simulink model "circuit5"  (Simulink 5.0)
settings: Solver=ode23tb  StartTime=0.0  StopTime=1  FixedStep=10e-6  RelTol=1e-4
undefined symbols (not defined in the file): A, powericon
libraries: powerlib2 x8, powerlib_extras x3, powerlib_models x1
settings Model: LastModifiedBy=Администратор

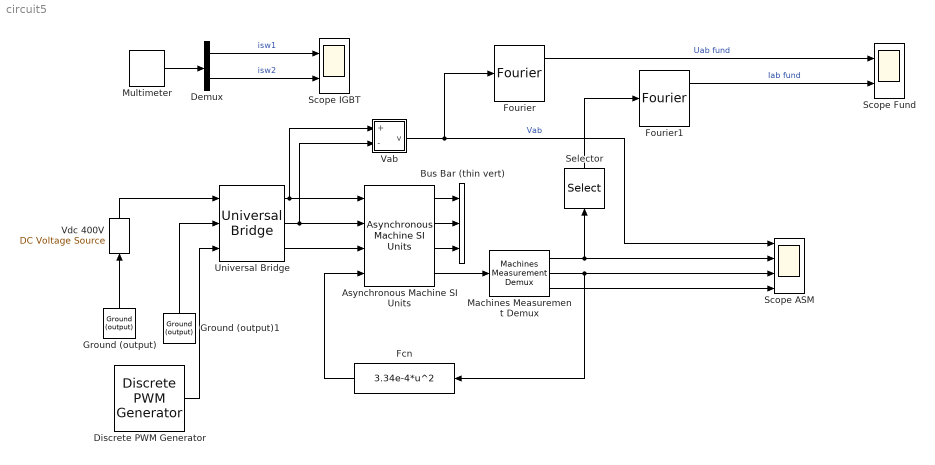
== system circuit5 ==
  Asynchronous Machine SI Units : powerlib2/Machines/Asynchronous Machine SI Units  Tag=PoWeRsYsTeMbLoCk  rotType=Wound  ctrl=Rotor  x1=[ 3*746, 220, 60 ]  x2="[ 0.435  2.0e-3 ]"  x3="[ 0.816  2.0e-3 ]"  x4=69.31e-3  x5="[ 0.089  0  2 ]"  x6="[ 1,0   0,0,0   0,0,0 ]"  PSBOutputType=1110  iounits=1  LoadFlowParameters=0
  Bus Bar (thin vert) : powerlib2/Connectors/Bus Bar (thin vert)  Tag=PoWeRsYsTeMbLoCk  input=3  output=0  PSBOutputType=111111111111111111111111111111111111111111111111111111111111111111111111111111111111
  Demux : Demux  Outputs=2
  Discrete PWM Generator : powerlib_extras/Discrete  Control Blocks/Discrete PWM Generator  GeneratorMode="3-arm  bridge (6 pulses)"  Fc=1080  Ts=10e-6  Internal=on  mIndex=0.9  Freq=60  Phase=0
  Fcn : Fcn  Orientation=left  Expr=3.34e-4*u^2
  Fourier : powerlib_extras/Measurements/Fourier  f1=60  n=1
  Fourier1 : powerlib_extras/Measurements/Fourier  f1=60  n=1
  Ground (output) : powerlib2/Connectors/Ground (output)  Tag=PoWeRsYsTeMbLoCk  Orientation=up  PSBOutputType=1
  Ground (output)1 : powerlib2/Connectors/Ground (output)  Tag=PoWeRsYsTeMbLoCk  Orientation=up  PSBOutputType=1
  Machines Measurement Demux : powerlib2/Machines/Machines Measurement Demux  machType=Asynchronous  ssm1=on  ssm2=on  ssm3=on  ssm4=on  ssm5=on  ssm6=on  sm1=on  sm2=off  sm3=off  sm4=off  sm5=off  sm6=off  sm7=off  sm8=on  sm9=off  sm10=off  sm11=off  sm115=on  sm12=off  sm13=off  sm14=off  asm1=off  asm2=off  asm3=off  asm4=off  asm5=on  asm6=off  asm7=off  asm8=off  asm9=on  asm10=on  asm11=off  pmsm1=on  pmsm2=on  pmsm3=on  pmsm4=on  pmsm5=on  pmsm6=on  lastType=1
  Multimeter : powerlib2/Measurements/Multimeter  Tag=PoWeRsYsTeMmEaSuReMeNt  PhasorSimulation=off  OutputType=Magnitude  sel=[1 2]  L=6  Gain=[1 1]  yselected={'Isw1: Universal Bridge','Isw2: Universal Bridge'};  PSBOutputType=1  PSBequivalent=0  AxesSetting=[0,0.1,-100,100]  Display=1  SavedBlockNames=-11
  Scope ASM : Scope  NumInputPorts=4
      settings: YMin=-500~-75~97.5~42.5  YMax=500~75~122.5~57.5
  Scope Fund : Scope  NumInputPorts=2
      settings: YMin=275~78  YMax=292.5~83
  Scope IGBT : Scope  NumInputPorts=2
      settings: YMin=-300~-200  YMax=292.5~200  SaveName=ScopeData2
  Selector : Selector  Orientation=up  InputPortWidth=3
  Universal Bridge : powerlib2/Power Electronics/Universal Bridge  Tag=PoWeRsYsTeMbLoCk  arms=3  confi=ABC as output terminals  injcc=1e5  cf=inf  device=IGBT / Diodes  Ron=1e-3  Lon=0  VFs="[  0  0  ]"  Vf=0  gtoparameters=[ 10e-6 , 20e-6 ]  igbtparameters=[ 1e-6 , 1e-6 ]  mesure=Device currents  PSBOutputType=111
  Vab : Subsystem  Tag=PoWeRsYsTeMmEaSuReMeNt  AncestorBlock=powerlib2/Measurements/Voltage Measurement  LoadFcn=powericon('psblcfmeas',gcb)  InitFcn=powericon('checksum',bdroot)  mask(Voltage Measurement){PhasorSimulation=off, OutputType=Magnitude, PSBOutputType=0, PSBequivalent=1}
      mask prompts: PhasorSimulation "Phasor simulation"; OutputType "Output signal :"; PSBOutputType "Output type [1=PSB  0=simulink output]"; PSBequivalent "Equivalent circuit"
      mask help: Ideal voltage measurement.
      mask init:
      | switch OutputType
      | case 1
      |     OutputSelection = 1;
      |     NormalMode = 2;
      |     PhasorMode = 1;
      | case 2
      |     OutputSelection =[2,3];
      |     NormalMode = 3;
      |     PhasorMode = [1,2];
      | case 3
      |     OutputSelection =[4,5];
      |     NormalMode = 3;
      |     PhasorMode = [1,2];
      | case 4
      |     OutputSelection =[4];
      |     NormalMode = 2;
      |     PhasorMode = 1;
      | end
      | %
      | if PhasorSimulation
      |     SelectionMode = PhasorMode;
      | else
      |     SelectionMode = NormalMode;
      | end
      settings: CopyFcn=powericon('psblcfmeas',gcb,1)  ModelCloseFcn=powericon('loadsavedata',gcs,'close')
      mask Help: web(psbhelp);
      mask StyleString: checkbox,popup(Complex|Real-Imag|Magnitude-Angle|Magnitude),edit,edit
  Vdc 400V : powerlib2/Electrical Sources/DC Voltage Source  Tag=PoWeRsYsTeMbLoCk  Description=source block  Orientation=up  V=400  mesure=None  PSBOutputType=1
  wires:
  Universal Bridge/1 -> Asynchronous Machine SI Units/1, Vab/1(+)
  Universal Bridge/2 -> Asynchronous Machine SI Units/2, Vab/2(-)
  Universal Bridge/3 -> Asynchronous Machine SI Units/3
  Asynchronous Machine SI Units/1 -> Bus Bar (thin vert)/1
  Asynchronous Machine SI Units/2 -> Bus Bar (thin vert)/2
  Asynchronous Machine SI Units/3 -> Bus Bar (thin vert)/3
  Asynchronous Machine SI Units/4 -> Machines Measurement Demux/1
  Machines Measurement Demux/2 -> Fcn/1, Scope ASM/3
  Fcn/1 -> Asynchronous Machine SI Units/4
  Vdc 400V/1 -> Universal Bridge/1
  Ground (output)/1 -> Vdc 400V/1
  Ground (output)1/1 -> Universal Bridge/2
  Discrete PWM Generator/1 -> Universal Bridge/3
  Vab/1(v) -> Fourier/1, Scope ASM/1  "Vab"
  Machines Measurement Demux/1 -> Selector/1, Scope ASM/2
  Selector/1 -> Fourier1/1
  Fourier/1 -> Scope Fund/1  "Uab fund"
  Fourier1/1 -> Scope Fund/2  "Iab fund"
  Machines Measurement Demux/3 -> Scope ASM/4
  Multimeter/1 -> Demux/1
  Demux/1 -> Scope IGBT/1  "isw1"
  Demux/2 -> Scope IGBT/2  "isw2"

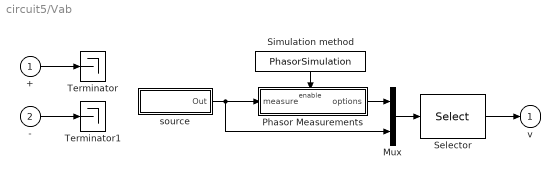
== system circuit5/Vab ==
  + : Inport
  - : Inport  Port=2
  Mux : Mux  Inputs=2
  Phasor Measurements : Subsystem  TreatAsAtomicUnit=on
  Selector : Selector  Elements=SelectionMode  InputPortWidth=length(OutputSelection)+1
  Simulation method : Constant  Orientation=down  Value=PhasorSimulation
  Terminator : Terminator
  Terminator1 : Terminator
  source : Subsystem
      mask init:
      | pss=powericon('loadsavedata','circuit5','load');if isempty(pss),A=0;B=0;C=0;D=0;x0=0;Rswitch=0;TypeSwitch=0;Ts=0;YSwitchCurrent=-1;else,A=pss.A;B=pss.B;C=pss.C;D=pss.D;x0=pss.x0;Rswitch=pss.Rswitch;TypeSwitch=pss.TypeSwitch;Ts=0;YSwitchCurrent=pss.YSwitchCurrent;end
  v : Outport  InitialOutput=0
  wires:
  source/1(Out) -> Phasor Measurements/1(measure), Mux/2
  +/1 -> Terminator/1
  -/1 -> Terminator1/1
  Selector/1 -> v/1
  Phasor Measurements/1(options) -> Mux/1
  Mux/1 -> Selector/1
  Simulation method/1 -> Phasor Measurements/Enable

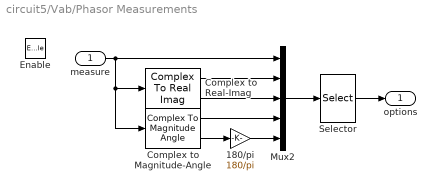
== system circuit5/Vab/Phasor Measurements ==
  measure : Inport
  Enable : EnablePort
  180/pi : Gain  Gain=180/pi  SaturateOnIntegerOverflow=on
  Complex to Magnitude-Angle : ComplexToMagnitudeAngle
  Complex to Real-Imag : ComplexToRealImag
  Mux2 : Mux  Inputs=5
  Selector : Selector  Elements=OutputSelection  InputPortWidth=5
  options : Outport  InitialOutput=0
  wires:
  Selector/1 -> options/1
  180/pi/1 -> Mux2/5
  Complex to Magnitude-Angle/2 -> 180/pi/1
  Complex to Magnitude-Angle/1 -> Mux2/4
  Complex to Real-Imag/2 -> Mux2/3
  Complex to Real-Imag/1 -> Mux2/2
  measure/1 -> Mux2/1, Complex to Real-Imag/1, Complex to Magnitude-Angle/1
  Mux2/1 -> Selector/1

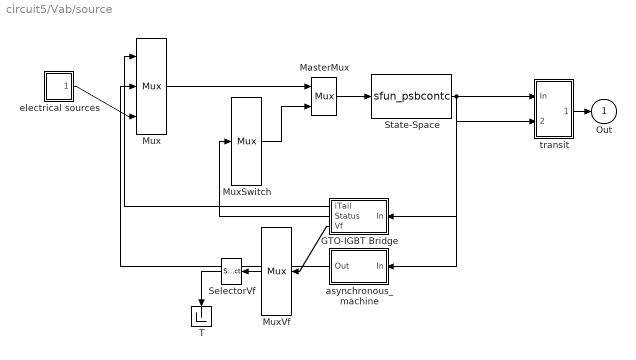
== system circuit5/Vab/source ==
  GTO-IGBT Bridge : Subsystem  Orientation=left
  MasterMux : Mux  Inputs=[-1 6]
  Mux : Mux  Inputs=[6 4 1]
  MuxSwitch : Mux  Inputs=1
  MuxVf : Mux  Orientation=left  Inputs=1
  SelectorVf : Selector  Orientation=left  InputPortWidth=6
  State-Space : S-Function  FunctionName=sfun_psbcontc  Parameters=A,B,C,D,x0,Rswitch,YSwitchCurrent
  T : Terminator
      settings: Orientation=down
  asynchronous_machine : Subsystem  Orientation=left
  electrical sources : Subsystem
  transit : Subsystem
  Out : Outport  InitialOutput=0
  wires:
  SelectorVf/1 -> T/1
  MuxVf/1 -> SelectorVf/1
  Mux/1 -> MasterMux/1
  MuxSwitch/1 -> MasterMux/2
  MasterMux/1 -> State-Space/1
  State-Space/1 -> transit/1(In), GTO-IGBT Bridge/1(In), asynchronous_machine/1(In), transit/2(signals)
  transit/1(Out) -> Out/1
  GTO-IGBT Bridge/1(iTail) -> Mux/1
  GTO-IGBT Bridge/2(Status) -> MuxSwitch/1
  GTO-IGBT Bridge/3(Vf) -> MuxVf/1
  asynchronous_machine/1(Out) -> Mux/2
  electrical sources/1(Out) -> Mux/3

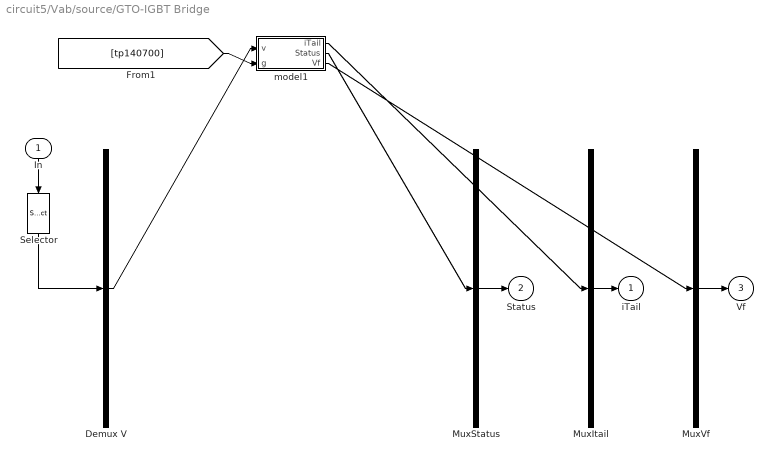
== system circuit5/Vab/source/GTO-IGBT Bridge ==
  In : Inport  Orientation=down
  Demux V : Demux  Outputs=1
  MuxItail : Mux  Inputs=1
  MuxStatus : Mux  Inputs=1
  MuxVf : Mux  Inputs=1
  Selector : Selector  Orientation=down  Elements=[1 2 3 4 5 6]  InputPortWidth=17
  model1 : Subsystem  AncestorBlock=powerlib_models/Continuous/GTO-IGBT Bridge  mask(GTO & IGBT Bridge Logic){nb_arm=3, Tf=1e-006, Tt=1e-006, Cs=Inf, VFs=[0 0], Rsw=0.001}
      mask prompts: nb_arm "Number of bridge arms (1,2 or 3)"; Tf "Curent 10% fall time Tf (s) :"; Tt "Current tail time Tt (s) :"; Cs "Snubber Capacitance Cs (F):"; VFs "Forward voltages [ Vf Vfd ]"; Rsw "Device resistances"
      mask help:
      | Generates the switch status ( 0 or 1) and the tail currents for a forced-commutated two- level bridge using GTO/Diode or IGBT/Diode pairs.
      | Specify  3 arms (6 switches) for 3 phase bridge, 2 arms for 4 switches, or 1 arm.
      | To turn-off the tail current, specify Tf=0 and Tt=0.
      mask init:
      | Vf=VFs(1);
      | Vfd=VFs(2);
      | nb_switch=nb_arm*2;
      | if nb_arm==1,
      |    Selec_Diode=[2 1];
      | elseif nb_arm==2,
      |    Selec_Diode=[2 1 4 3];
      | elseif nb_arm==3,
      |    Selec_Diode=[2 1 4 3 6 5];
      | end
  iTail : Outport  InitialOutput=0
  Status : Outport  Port=2  InitialOutput=0
  Vf : Outport  Port=3  InitialOutput=0
  wires:
  Selector/1 -> Demux V/1
  In/1 -> Selector/1
  MuxVf/1 -> Vf/1
  MuxItail/1 -> iTail/1
  MuxStatus/1 -> Status/1
  model1/1(iTail) -> MuxItail/1
  Demux V/1 -> model1/1("v ")
  model1/2(Status) -> MuxStatus/1
  model1/3(Vf) -> MuxVf/1
  [tp140700] -> model1/2(g)

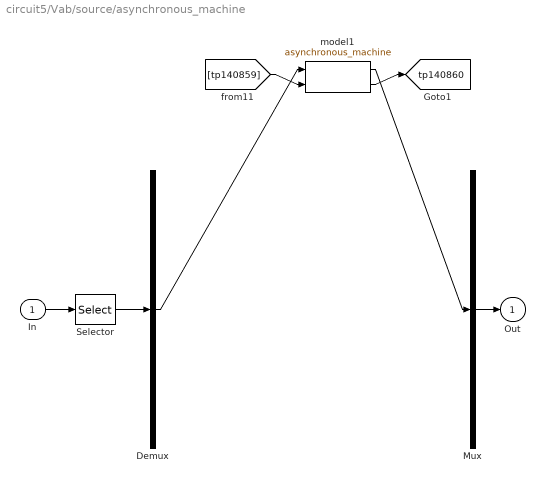
== system circuit5/Vab/source/asynchronous_machine ==
  In : Inport
  Demux : Demux  Outputs=1
  Mux : Mux  Inputs=1
  Selector : Selector  Elements=[7 8 9 10]  InputPortWidth=17
  model1 : powerlib_models/Continuous/asynchronous_machine  rotType=Wound  ctrl=Rotor  nom=[2238 220 60]  sta=[0.0201142561983471 0.0348638893821519]  rot=[0.0377315702479339 0.0348638893821519]  Lm=1.20820808653847  mec=[0.706483746673152 0 2]  ini=[1 0 0 0 0 0 0 0]  iounits=on
  Out : Outport  InitialOutput=0
  tag scope: tp140860=global
  wires:
  Mux/1 -> Out/1
  Selector/1 -> Demux/1
  In/1 -> Selector/1
  Demux/1 -> model1/1
  model1/1 -> Mux/1
  model1/2 -> [tp140860]
  [tp140859] -> model1/2

== system circuit5/Vab/source/electrical sources ==
  Mux : Mux  Inputs=[-1]
  Selector : Selector  InputPortWidth=2
  Out : Outport  InitialOutput=0
  wires:
  Selector/1 -> Out/1
  Mux/1 -> Selector/1
  [tp140629] -> Mux/1

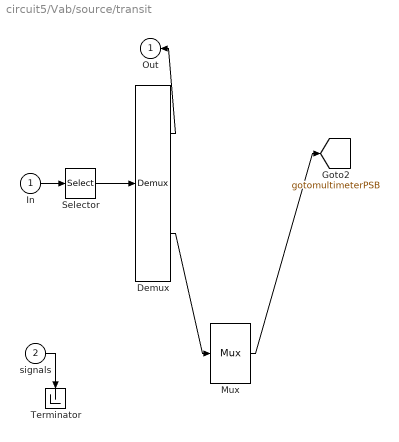
== system circuit5/Vab/source/transit ==
  In : Inport
  signals : Inport  Port=2
  Demux : Demux  Outputs=[1 6]
  Mux : Mux  Inputs=1
  Selector : Selector  Elements=[11 12 13 14 15 16 17]  InputPortWidth=17
  Terminator : Terminator
      settings: Orientation=down
  Out : Outport  Orientation=left  InitialOutput=0
  tag scope: gotomultimeterPSB=global
  wires:
  signals/1 -> Terminator/1
  Selector/1 -> Demux/1
  In/1 -> Selector/1
  Demux/1 -> Out/1
  Demux/2 -> Mux/1
  Mux/1 -> [gotomultimeterPSB]

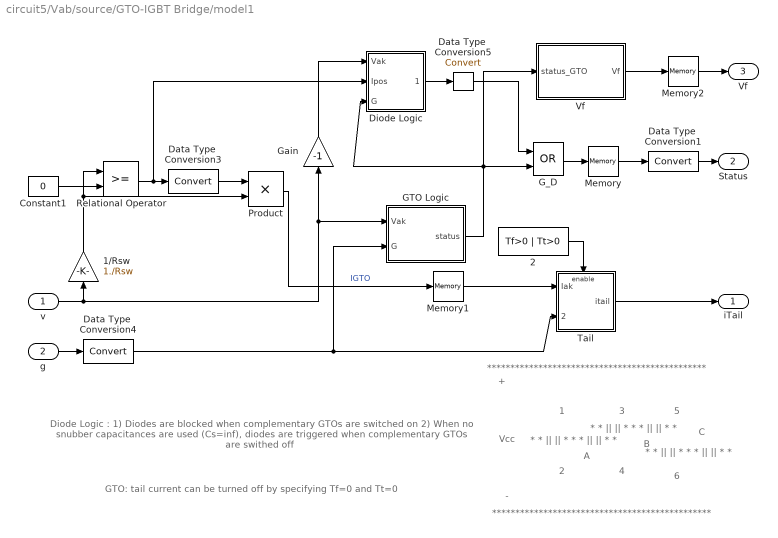
== system circuit5/Vab/source/GTO-IGBT Bridge/model1 ==
  note: *
      | *
      | ||
      | ||
      | *
      | *
      | *
      | ||
      | ||
      | *
      | *
  note: 1
  note: 2
  note: +
  note: -
  note: *
      | *
      | ||
      | ||
      | *
      | *
      | *
      | ||
      | ||
      | *
      | *
  note: 3
  note: 4
  note: ***********************************************
  note: Vcc
  note: A
  note: B
  note: *
      | *
      | ||
      | ||
      | *
      | *
      | *
      | ||
      | ||
      | *
      | *
  note: C
  note: ***********************************************
  note: 5
  note: 6
  note: Diode Logic :
      | 1) Diodes are blocked when complementary GTOs are switched on
      | 2) When no snubber capacitances are used (Cs=inf), diodes are triggered
      | when complementary GTOs are swithed off
  note: GTO:
      |  tail current can be turned off by specifying Tf=0 and Tt=0
  "v " : Inport
  g : Inport  Port=2
  1/Rsw : Gain  Orientation=up  Gain=1./Rsw  SaturateOnIntegerOverflow=on
  2 : Constant  Value=Tf>0 | Tt>0
  Constant1 : Constant  Value=0
  Data Type  Conversion1 : DataTypeConversion  DataType=double  SaturateOnIntegerOverflow=on
  Data Type  Conversion3 : DataTypeConversion  DataType=double  SaturateOnIntegerOverflow=on
  Data Type  Conversion4 : DataTypeConversion  DataType=boolean  SaturateOnIntegerOverflow=on
  Data Type  Conversion5 : DataTypeConversion  DataType=boolean  SaturateOnIntegerOverflow=on
  Diode Logic : Subsystem
  GTO Logic : Subsystem
  G_D : Logic  Operator=OR
  Gain : Gain  Orientation=up  Gain=-1  SaturateOnIntegerOverflow=on
  Memory : Memory  InheritSampleTime=on
  Memory1 : Memory  InheritSampleTime=on
  Memory2 : Memory  InheritSampleTime=on
  Product : Product  SaturateOnIntegerOverflow=on  InputSameDT=on
  Relational Operator : RelationalOperator  InputSameDT=on
  "Tail " : Subsystem  TreatAsAtomicUnit=on  mask(Gto tail current){Tf=Tf, Tt=Tt}
      mask prompts: Tf "Current 10% fall time Tf (s) :"; Tt "Current tail time Tt (s) :"
  "Vf " : Subsystem
  iTail : Outport
  Status : Outport  Port=2
  Vf : Outport  Port=3
  wires:
  1/Rsw/1 -> Product/2, Relational Operator/1
  Data Type  Conversion5/1 -> G_D/1
  Diode Logic/1(status) -> Data Type  Conversion5/1
  Data Type  Conversion4/1 -> GTO Logic/2(G), "Tail "/2(switch)
  g/1 -> Data Type  Conversion4/1
  Relational Operator/1 -> Diode Logic/2(Ipos), Data Type  Conversion3/1
  Data Type  Conversion3/1 -> Product/1
  Data Type  Conversion1/1 -> Status/1
  Memory/1 -> Data Type  Conversion1/1
  Product/1 -> Memory1/1  "IGTO"
  Gain/1 -> Diode Logic/1(Vak)
  Memory1/1 -> "Tail "/1(Iak)
  Constant1/1 -> Relational Operator/2
  G_D/1 -> Memory/1
  2/1 -> "Tail "/Enable
  "Tail "/1(itail) -> iTail/1
  "v "/1 -> 1/Rsw/1, GTO Logic/1(Vak), Gain/1
  "Vf "/1(Vf) -> Memory2/1
  GTO Logic/1(status) -> G_D/2, Diode Logic/3(G), "Vf "/1(status_GTO)
  Memory2/1 -> Vf/1

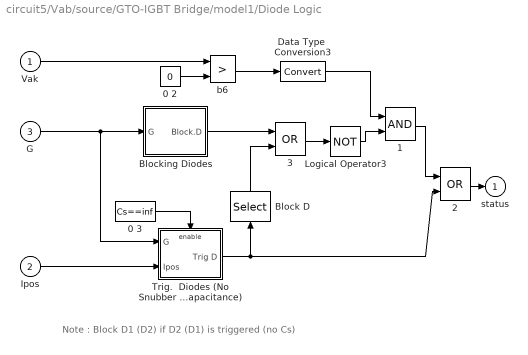
== system circuit5/Vab/source/GTO-IGBT Bridge/model1/Diode Logic ==
  note: Note : Block D1 (D2) if D2 (D1) is triggered (no Cs)
  Vak : Inport
  Ipos : Inport  Port=2
  G : Inport  Port=3
  0 2 : Constant  Value=0
  0 3 : Constant  Value=Cs==inf
  1 : Logic
  2 : Logic  Operator=OR
  3 : Logic  Operator=OR
  Block D : Selector  Orientation=up  Elements=Selec_Diode  InputPortWidth=nb_switch
  Blocking Diodes : Subsystem
  Data Type  Conversion3 : DataTypeConversion  DataType=boolean  SaturateOnIntegerOverflow=on
  Logical Operator3 : Logic  Operator=NOT
  Trig.  Diodes (No Snubber Capacitance) : Subsystem  TreatAsAtomicUnit=on
  b6 : RelationalOperator  Operator=>  InputSameDT=on
  status : Outport  InitialOutput=0
  wires:
  Data Type  Conversion3/1 -> 1/1
  b6/1 -> Data Type  Conversion3/1
  Block D/1 -> 3/2
  Trig.  Diodes (No Snubber Capacitance)/1(Trig D) -> Block D/1, 2/2
  3/1 -> Logical Operator3/1
  Logical Operator3/1 -> 1/2
  1/1 -> 2/1
  2/1 -> status/1
  Blocking Diodes/1(Block.D) -> 3/1
  Vak/1 -> b6/1
  0 2/1 -> b6/2
  G/1 -> Blocking Diodes/1(G), Trig.  Diodes (No Snubber Capacitance)/1(G)
  Ipos/1 -> Trig.  Diodes (No Snubber Capacitance)/2(Ipos)
  0 3/1 -> Trig.  Diodes (No Snubber Capacitance)/Enable

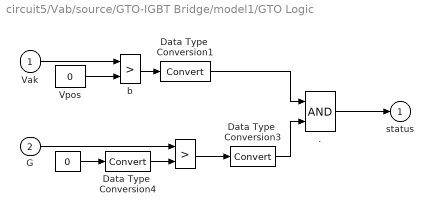
== system circuit5/Vab/source/GTO-IGBT Bridge/model1/GTO Logic ==
  Vak : Inport
  G : Inport  Port=2
  " " : RelationalOperator  Operator=>  InputSameDT=on
  "    " : Constant  Value=0
  ". " : Logic
  Data Type  Conversion1 : DataTypeConversion  DataType=boolean  SaturateOnIntegerOverflow=on
  Data Type  Conversion3 : DataTypeConversion  DataType=boolean  SaturateOnIntegerOverflow=on
  Data Type  Conversion4 : DataTypeConversion  DataType=boolean  SaturateOnIntegerOverflow=on
  Vpos : Constant  Value=0
  b : RelationalOperator  Operator=>  InputSameDT=on
  status : Outport  InitialOutput=0
  wires:
  Data Type  Conversion4/1 -> " "/2
  "    "/1 -> Data Type  Conversion4/1
  Data Type  Conversion3/1 -> ". "/2
  " "/1 -> Data Type  Conversion3/1
  Data Type  Conversion1/1 -> ". "/1
  b/1 -> Data Type  Conversion1/1
  G/1 -> " "/1
  Vpos/1 -> b/2
  Vak/1 -> b/1
  ". "/1 -> status/1

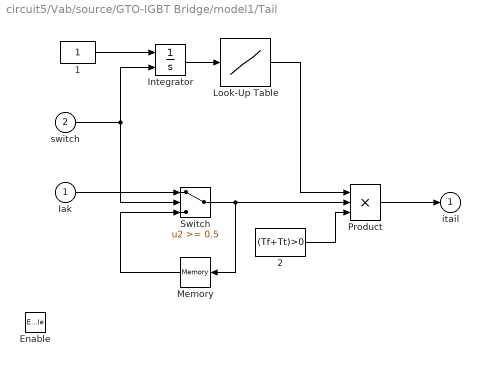
== system circuit5/Vab/source/GTO-IGBT Bridge/model1/Tail  ==
  Iak : Inport
  switch : Inport  Port=2
  Enable : EnablePort  StatesWhenEnabling=reset
  1 : Constant
  2 : Constant  Value=(Tf+Tt)>0  ShowAdditionalParam=on  OutDataTypeMode=double
  Integrator : Integrator  ExternalReset=falling
  Look-Up Table : Lookup  InputValues="[  0   Tf+eps Tf+Tt+2*eps  Tf+Tt+3*eps]"  OutputValues="[  1   0.1*(Tt>0) 0 0]"  SaturateOnIntegerOverflow=on
  Memory : Memory  Orientation=left  InheritSampleTime=on
  Product : Product  Inputs=3  SaturateOnIntegerOverflow=on  InputSameDT=on
  Switch : Switch  Threshold=0.5  InputSameDT=on
  itail : Outport  InitialOutput=0
  wires:
  Memory/1 -> Switch/3
  Switch/1 -> Memory/1, Product/2
  Product/1 -> itail/1
  Integrator/1 -> Look-Up Table/1
  switch/1 -> Integrator/2, Switch/2
  Iak/1 -> Switch/1
  1/1 -> Integrator/1
  Look-Up Table/1 -> Product/1
  2/1 -> Product/3

== system circuit5/Vab/source/GTO-IGBT Bridge/model1/Vf  ==
  status_GTO : Inport
  Switch : Switch  Threshold=0.5  InputSameDT=on
  Vf device : Constant  Value=Vf*ones(nb_switch,1)
  Vf diode : Constant  Value=-Vfd*ones(nb_switch,1)
  Vf : Outport  InitialOutput=[0]
  wires:
  Vf device/1 -> Switch/1
  Vf diode/1 -> Switch/3
  Switch/1 -> Vf/1
  status_GTO/1 -> Switch/2

== system circuit5/Vab/source/GTO-IGBT Bridge/model1/Diode Logic/Blocking Diodes ==
  G : Inport
  Bloque D214365 : Selector  Elements=Selec_Diode  InputPortWidth=nb_switch
  Logical Operator : Logic  Operator=NOT
  Memory : Memory  InheritSampleTime=on
  Pulse 1 step : Logic
  Block.D : Outport
  wires:
  G/1 -> Pulse 1 step/2, Memory/1
  Logical Operator/1 -> Pulse 1 step/1
  Memory/1 -> Logical Operator/1
  Pulse 1 step/1 -> Bloque D214365/1  "Blockinkg"
  Bloque D214365/1 -> Block.D/1

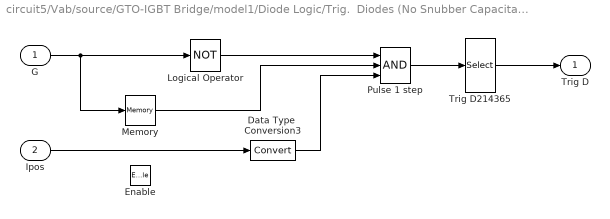
== system circuit5/Vab/source/GTO-IGBT Bridge/model1/Diode Logic/Trig.  Diodes (No Snubber Capacitance) ==
  G : Inport
  Ipos : Inport  Port=2
  Enable : EnablePort  StatesWhenEnabling=reset
  Data Type  Conversion3 : DataTypeConversion  DataType=boolean  SaturateOnIntegerOverflow=on
  Logical Operator : Logic  Operator=NOT
  Memory : Memory  InheritSampleTime=on
  Pulse 1 step : Logic  Inputs=3
  Trig D214365 : Selector  Elements=Selec_Diode  InputPortWidth=nb_switch
  Trig D : Outport
  wires:
  Data Type  Conversion3/1 -> Pulse 1 step/3
  Ipos/1 -> Data Type  Conversion3/1
  G/1 -> Logical Operator/1, Memory/1
  Logical Operator/1 -> Pulse 1 step/1
  Memory/1 -> Pulse 1 step/2
  Pulse 1 step/1 -> Trig D214365/1
  Trig D214365/1 -> Trig D/1
